simulink model "robot"  (R2022a)
settings: Solver=VariableStepAuto  StartTime=0.0  StopTime=10.0  RelTol=1e-3
undefined symbols (not defined in the file): A, B, C, D, Ki, Kx, l, L
settings Model: Creator=fduterte  LastModifiedBy=Amandine
settings SolverCC: AlgebraicLoopSolver=TrustRegion
settings DebuggingCC: UnconnectedInputMsg=warning  UnconnectedOutputMsg=warning  UnconnectedLineMsg=warning  SFMachineParentedDataDiag=warning
settings RTWCC: DLArmComputeVersion=19.05

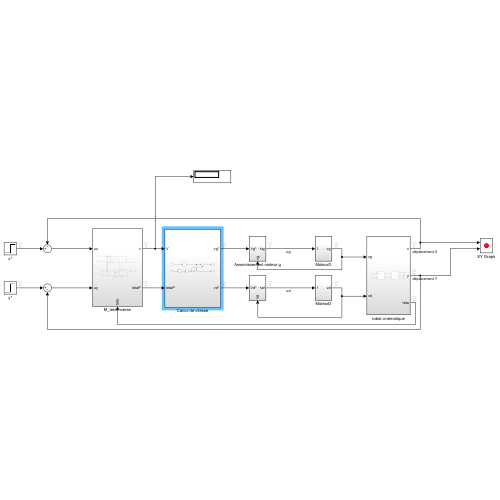
[thumbnail: Simulink's stored preview of the top-level diagram]
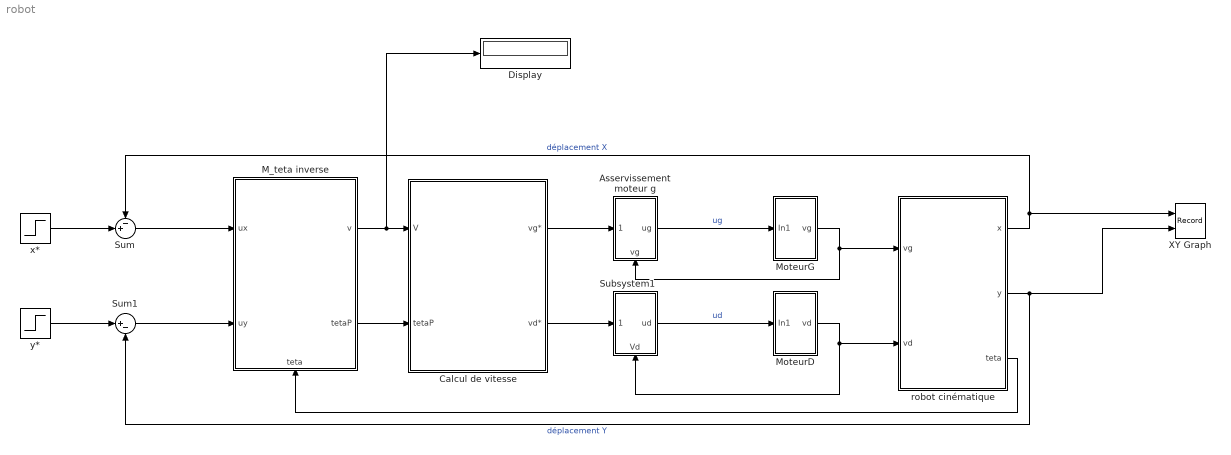
== system robot ==
  Asservissement moteur g : Subsystem
      settings: PortSchema="{\"entries\":[{\"content\":{\"sides\":[{\"content\":{\"connectorIds\":[\"In1\"]},\"type\":\"ConnectorPlacement.EquallySpacedRectSide\",\"uuid\":\"974f67ff-ec86-461c-aa60-533cdeafb118\"},{\"content\":{\"connectorIds\":[\"Out1\"],\"side\":\"RIGHT\"},\"type\":\"ConnectorPlacement.EquallySpacedRectSide\",\"uuid\":\"c8387546-9b25-43fb-a7e6-791e04dec918\"},{\"content\":{\"connectorIds\":[],\"side\":\"TOP\"},\"type\":\"ConnectorPlacement.EquallySpacedRectSide\",\"uuid\":\"89b9c1e4-8a21-45f2-bc89-d00f29d45e47\"},{\"content\":{\"connectorIds\":[\"In2\"],\"side\":\"BOTTOM\"},\"type\":\"ConnectorPlacement.EquallySpacedRectSide\",\"uuid\":\"53d6fe91-d338-4930-b8cd-dea5889de835\"},{\"content\":{\"connectorIds\":[],\"side\":\"HIDDEN\"},\"type\":\"ConnectorPlacement.EquallySpacedRectSide\",\"uuid\":\"29b397e1-e792-4e18-a134-a46f0e718b0f\"}]},\"type\":\"ConnectorPlacement.EquallySpacedConnector\",\"uuid\":\"81d111f1-5eeb-4176-9ac3-35ecafc98cd8\"}],\"packageUris\":[\"http://schema.mathworks.com/mf0/Connector/R2020b\"],\"version\":\"1.0\"}"
  Calcul de vitesse : Subsystem
  Display : Display
  M_teta inverse : Subsystem
      settings: PortSchema="{\"entries\":[{\"content\":{\"sides\":[{\"content\":{\"connectorIds\":[\"In1\",\"In2\"]},\"type\":\"ConnectorPlacement.EquallySpacedRectSide\",\"uuid\":\"46188908-b1cc-4882-9b8e-a8476c333113\"},{\"content\":{\"connectorIds\":[\"Out1\",\"Out2\"],\"side\":\"RIGHT\"},\"type\":\"ConnectorPlacement.EquallySpacedRectSide\",\"uuid\":\"d9e3f140-d678-4bcd-b58f-e0cf2d32dddf\"},{\"content\":{\"connectorIds\":[],\"side\":\"TOP\"},\"type\":\"ConnectorPlacement.EquallySpacedRectSide\",\"uuid\":\"a6a59054-5aa4-4aac-8c2f-440078fd31e6\"},{\"content\":{\"connectorIds\":[\"In3\"],\"side\":\"BOTTOM\"},\"type\":\"ConnectorPlacement.EquallySpacedRectSide\",\"uuid\":\"d37c5d7c-eb10-4efc-bec5-b12ca0db436e\"},{\"content\":{\"connectorIds\":[],\"side\":\"HIDDEN\"},\"type\":\"ConnectorPlacement.EquallySpacedRectSide\",\"uuid\":\"27b7b574-64a3-4ae5-a49b-592b93501c4d\"}]},\"type\":\"ConnectorPlacement.EquallySpacedConnector\",\"uuid\":\"41e6c7f6-3ce7-4034-83c9-1a8b5fe3dc83\"}],\"packageUris\":[\"http://schema.mathworks.com/mf0/Connector/R2020b\"],\"version\":\"1.0\"}"
  MoteurD : Subsystem
  MoteurG : Subsystem
  Subsystem1 : Subsystem
      settings: PortSchema="{\"entries\":[{\"content\":{\"sides\":[{\"content\":{\"connectorIds\":[\"In1\"]},\"type\":\"ConnectorPlacement.EquallySpacedRectSide\",\"uuid\":\"974f67ff-ec86-461c-aa60-533cdeafb118\"},{\"content\":{\"connectorIds\":[\"Out1\"],\"side\":\"RIGHT\"},\"type\":\"ConnectorPlacement.EquallySpacedRectSide\",\"uuid\":\"c8387546-9b25-43fb-a7e6-791e04dec918\"},{\"content\":{\"connectorIds\":[],\"side\":\"TOP\"},\"type\":\"ConnectorPlacement.EquallySpacedRectSide\",\"uuid\":\"89b9c1e4-8a21-45f2-bc89-d00f29d45e47\"},{\"content\":{\"connectorIds\":[\"In2\"],\"side\":\"BOTTOM\"},\"type\":\"ConnectorPlacement.EquallySpacedRectSide\",\"uuid\":\"920a09e2-1f74-455c-9562-9225d36fe6fa\"},{\"content\":{\"connectorIds\":[],\"side\":\"HIDDEN\"},\"type\":\"ConnectorPlacement.EquallySpacedRectSide\",\"uuid\":\"29b397e1-e792-4e18-a134-a46f0e718b0f\"}]},\"type\":\"ConnectorPlacement.EquallySpacedConnector\",\"uuid\":\"81d111f1-5eeb-4176-9ac3-35ecafc98cd8\"}],\"packageUris\":[\"http://schema.mathworks.com/mf0/Connector/R2020b\"],\"version\":\"1.0\"}"
  Sum : Sum  Inputs=-+|
  Sum1 : Sum  Inputs=|+-
  XY Graph : Record  FileSettingsInternal="{\"entries\":[{\"content\":{\"excelSettings\":{\"content\":{},\"type\":\"Streamout.ExcelSettings\"}},\"type\":\"Streamout.FileSettingStorage\",\"uuid\":\"d9b7ccbf-8b1c-4774-986d-cf4be9a417a1\"}],\"packageUris\":[\"http://schema.mathworks.com/mf0/streamout_blocks/R2020a\"],\"version\":\"1.0\"}"  Layout=[1 1]  SignalsInternal="{\"entries\":[{\"content\":{\"signals\":[{\"content\":{\"blockPath\":[\"robot/XY Graph\"],\"channel\":[],\"dimensions\":[1],\"domain\":\"robot/XY Graph\",\"lineColor\":\"#a2142f\",\"plots\":[1],\"port\":1,\"sid\":[],\"signalID\":17,\"signalName\":\"XY Graph:1\"},\"type\":\"RecordBlkView.Signal\",\"uuid\":\"e619f21a-7836-4c61-a051-832b143e0227\"},{\"content\":{\"blockPath\":[\"robot/XY Graph\"],\"channel\":[],\"dimensions\":[1],\"domain\":\"robot/XY Graph\",\"lineColor\":\"#139fff\",\"plots\":[1],\"port\":2,\"sid\":[],\"signalID\":20,\"signalName\":\"XY Graph:2\"},\"type\":\"RecordBlkView.Signal\",\"uuid\":\"4c19a49e-2d7a-439d-9925-7ed591ba5977\"}]},\"type\":\"RecordBlkView.InputSignals\",\"uuid\":\"d8d664c2-0254-4fe2-9c50-e0796b544cb5\"}],\"packageUris\":[\"http://schema.mathworks.com/mf0/streamout_blocks/R2020a\"],\"version\":\"1.0\"}"  VisualizationBindings="{\"xyplotplugin\":{\"info\":[{\"series\":[{\"bindingParametersList\":[{\"parameter\":\"X-Axis\",\"signalID\":17,\"signalName\":\"XY Graph:1\"},{\"parameter\":\"Y-Axis\",\"signalID\":20,\"signalName\":\"XY Graph:2\"}],\"seriesID\":55674}],\"subplotID\":1}]}}"  CompatibilityTag=XY  st=-1
  robot cinématique : Subsystem
  x* : Step  After=1000  SampleTime=0
  y* : Step  After=500  SampleTime=0
  wires:
  x*/1 -> Sum/2
  robot cinématique/2(y) -> XY Graph/2, Sum1/2  "déplacement Y"
  robot cinématique/3(teta) -> M_teta inverse/3(teta)
  Sum1/1 -> M_teta inverse/2(uy)
  robot cinématique/1(x) -> XY Graph/1, Sum/1  "déplacement X"
  Asservissement moteur g/1(ug) -> MoteurG/1(In1)  "ug"
  MoteurG/1(vg) -> robot cinématique/1(vg), Asservissement moteur g/2(vg)
  MoteurD/1(vd) -> robot cinématique/2(vd), Subsystem1/2(Vd)
  Sum/1 -> M_teta inverse/1(ux)
  Subsystem1/1(ud) -> MoteurD/1(In1)  "ud"
  Calcul de vitesse/1(vg*) -> Asservissement moteur g/1(Vg*)
  Calcul de vitesse/2(vd*) -> Subsystem1/1(Vd*)
  M_teta inverse/1(v) -> Display/1, Calcul de vitesse/1(V)
  M_teta inverse/2(tetaP) -> Calcul de vitesse/2(tetaP)
  y*/1 -> Sum1/1

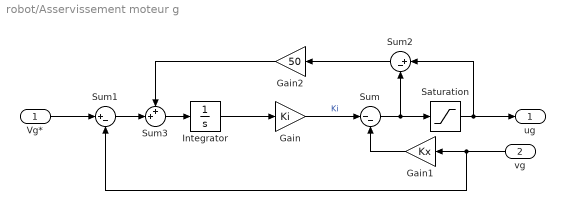
== system robot/Asservissement moteur g ==
  Vg* : Inport
  vg : Inport  Port=2
  Gain : Gain  Gain=Ki
  Gain1 : Gain  Gain=Kx
  Gain2 : Gain  Gain=50
  Integrator : Integrator
  Saturation : Saturate  UpperLimit=9  LowerLimit=-9
  Sum : Sum  Inputs=|--
  Sum1 : Sum  Inputs=|+-
  Sum2 : Sum  Inputs=|+-
  Sum3 : Sum  Inputs=++|
  ug : Outport
  wires:
  Integrator/1 -> Gain/1
  Gain/1 -> Sum/1  "Ki"
  Vg*/1 -> Sum1/1
  Gain1/1 -> Sum/2
  vg/1 -> Sum1/2, Gain1/1
  Sum1/1 -> Sum3/2
  Sum3/1 -> Integrator/1
  Sum2/1 -> Gain2/1
  Saturation/1 -> Sum2/1, ug/1
  Sum/1 -> Sum2/2, Saturation/1
  Gain2/1 -> Sum3/1

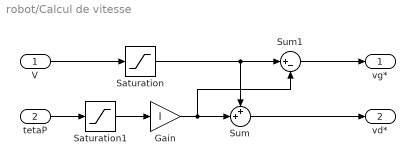
== system robot/Calcul de vitesse ==
  V : Inport
  tetaP : Inport  Port=2
  Gain : Gain  Gain=l
  Saturation : Saturate  UpperLimit=300  LowerLimit=-300
  Saturation1 : Saturate  UpperLimit=300/l  LowerLimit=-300/l
  Sum : Sum  Inputs=++|
  Sum1 : Sum  Inputs=|+-
  vg* : Outport
  vd* : Outport  Port=2
  wires:
  tetaP/1 -> Saturation1/1
  V/1 -> Saturation/1
  Gain/1 -> Sum1/2, Sum/2
  Sum/1 -> vd*/1
  Sum1/1 -> vg*/1
  Saturation/1 -> Sum1/1, Sum/1
  Saturation1/1 -> Gain/1

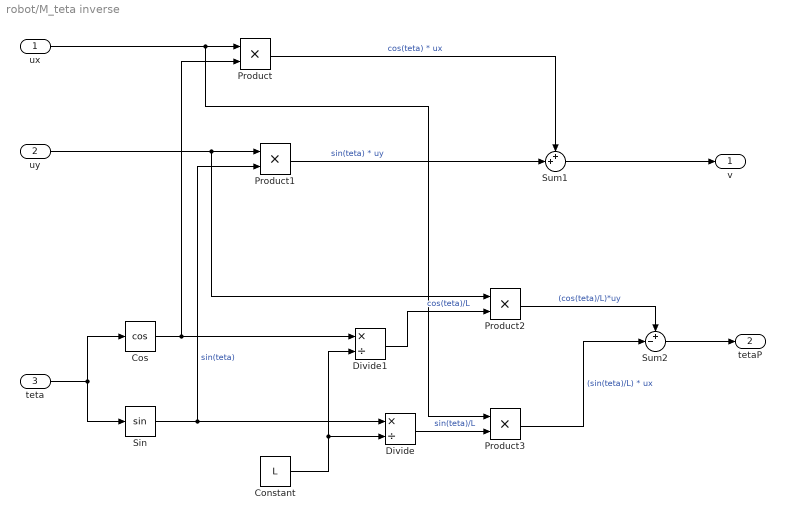
== system robot/M_teta inverse ==
  ux : Inport
  uy : Inport  Port=2
  teta : Inport  Port=3
  Constant : Constant  Value=L
  Cos : Trigonometry  Operator=cos
  Divide : Product  Inputs=*/
  Divide1 : Product  Inputs=*/
  Product{,1..3} (4 alike) : Product
  Sin : Trigonometry
  Sum1 : Sum  Inputs=++|
  Sum2 : Sum  Inputs=+-|
  v : Outport
  tetaP : Outport  Port=2
  wires:
  teta/1 -> Cos/1, Sin/1
  Cos/1 -> Product/2, Divide1/1
  Product1/1 -> Sum1/2  "sin(teta) * uy"
  Sum2/1 -> tetaP/1
  Sum1/1 -> v/1
  ux/1 -> Product3/1, Product/1
  Product/1 -> Sum1/1  "cos(teta) * ux"
  uy/1 -> Product2/1, Product1/1
  Sin/1 -> Divide/1, Product1/2  "sin(teta)"
  Constant/1 -> Divide1/2, Divide/2
  Divide1/1 -> Product2/2  "cos(teta)/L"
  Divide/1 -> Product3/2  "sin(teta)/L"
  Product3/1 -> Sum2/2  "(sin(teta)/L) * ux"
  Product2/1 -> Sum2/1  "(cos(teta)/L)*uy"

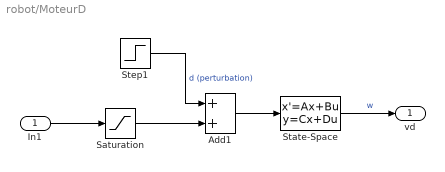
== system robot/MoteurD ==
  In1 : Inport
  Add1 : Sum
  Saturation : Saturate  UpperLimit=9  LowerLimit=-9
  State-Space : StateSpace  A=A  B=B  C=C  D=D  InitialCondition=0
  Step1 : Step  Time=5  After=0  SampleTime=0
  vd : Outport
  wires:
  Step1/1 -> Add1/1  "d (perturbation)"
  Add1/1 -> State-Space/1
  In1/1 -> Saturation/1
  State-Space/1 -> vd/1  "w"
  Saturation/1 -> Add1/2

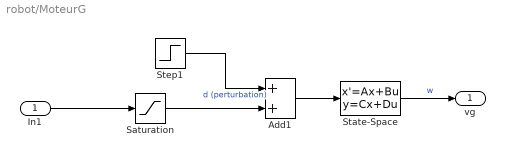
== system robot/MoteurG ==
  In1 : Inport
  Add1 : Sum
  Saturation : Saturate  UpperLimit=9  LowerLimit=-9
  State-Space : StateSpace  A=A  B=B  C=C  D=D  InitialCondition=0
  Step1 : Step  Time=5  After=0  SampleTime=0
  vg : Outport
  wires:
  Step1/1 -> Add1/1  "d (perturbation)"
  Add1/1 -> State-Space/1
  In1/1 -> Saturation/1
  State-Space/1 -> vg/1  "w"
  Saturation/1 -> Add1/2

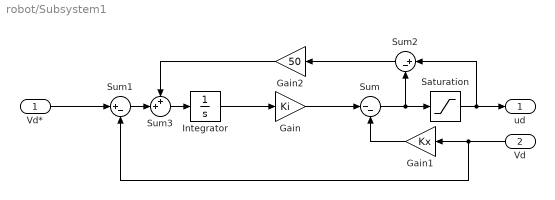
== system robot/Subsystem1 ==
  Vd* : Inport
  Vd : Inport  Port=2
  Gain : Gain  Gain=Ki
  Gain1 : Gain  Gain=Kx
  Gain2 : Gain  Gain=50
  Integrator : Integrator
  Saturation : Saturate  UpperLimit=9  LowerLimit=-9
  Sum : Sum  Inputs=|--
  Sum1 : Sum  Inputs=|+-
  Sum2 : Sum  Inputs=|+-
  Sum3 : Sum  Inputs=++|
  ud : Outport
  wires:
  Integrator/1 -> Gain/1
  Gain/1 -> Sum/1
  Vd*/1 -> Sum1/1
  Gain1/1 -> Sum/2
  Vd/1 -> Sum1/2, Gain1/1
  Sum1/1 -> Sum3/2
  Sum3/1 -> Integrator/1
  Sum2/1 -> Gain2/1
  Sum/1 -> Sum2/2, Saturation/1
  Saturation/1 -> Sum2/1, ud/1
  Gain2/1 -> Sum3/1

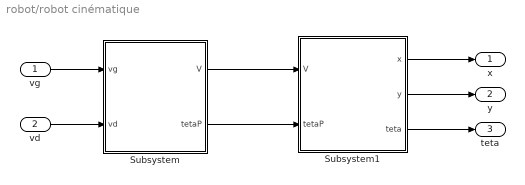
== system robot/robot cinématique ==
  vg : Inport
  vd : Inport  Port=2
  Subsystem : Subsystem
  Subsystem1 : Subsystem
  x : Outport
  y : Outport  Port=2
  teta : Outport  Port=3
  wires:
  Subsystem1/2(y) -> y/1
  Subsystem1/1(x) -> x/1
  Subsystem1/3(teta) -> teta/1
  Subsystem/1(V) -> Subsystem1/1(V)
  Subsystem/2(tetaP) -> Subsystem1/2(tetaP)
  vd/1 -> Subsystem/2(vd)
  vg/1 -> Subsystem/1(vg)

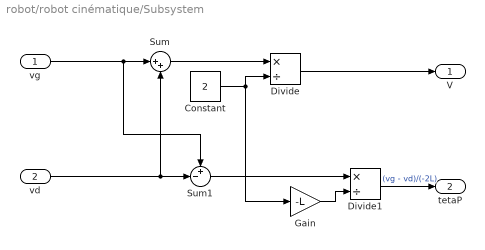
== system robot/robot cinématique/Subsystem ==
  vg : Inport
  vd : Inport  Port=2
  Constant : Constant  Value=2
  Divide : Product  Inputs=*/
  Divide1 : Product  Inputs=*/
  Gain : Gain  Gain=-L
  Sum : Sum  Inputs=|++
  Sum1 : Sum  Inputs=+-|
  V : Outport
  tetaP : Outport  Port=2
  wires:
  vg/1 -> Sum1/1, Sum/1
  vd/1 -> Sum1/2, Sum/2
  Sum/1 -> Divide/1
  Constant/1 -> Gain/1, Divide/2
  Divide/1 -> V/1
  Sum1/1 -> Divide1/1
  Divide1/1 -> tetaP/1  "(vg - vd)/(-2L)"
  Gain/1 -> Divide1/2

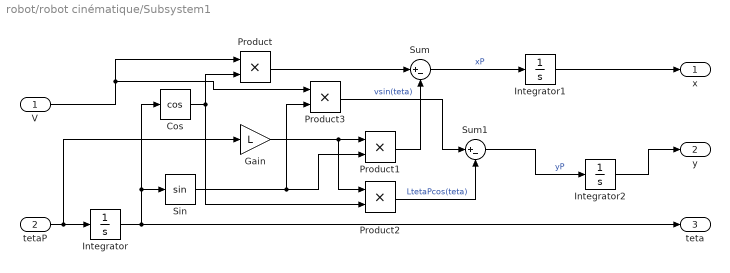
== system robot/robot cinématique/Subsystem1 ==
  V : Inport
  tetaP : Inport  Port=2
  Cos : Trigonometry  Operator=cos
  Gain : Gain  Gain=L
  Integrator : Integrator
  Integrator1 : Integrator
  Integrator2 : Integrator
  Product{,1..3} (4 alike) : Product
  Sin : Trigonometry
  Sum : Sum  Inputs=|+-
  Sum1 : Sum  Inputs=|+-
  x : Outport
  y : Outport  Port=2
  teta : Outport  Port=3
  wires:
  Integrator/1 -> teta/1, Sin/1, Cos/1
  tetaP/1 -> Integrator/1, Gain/1
  V/1 -> Product/1, Product3/1
  Cos/1 -> Product2/2, Product/2
  Product/1 -> Sum/1
  Gain/1 -> Product2/1, Product1/1
  Sin/1 -> Product3/2, Product1/2
  Product1/1 -> Sum/2
  Sum/1 -> Integrator1/1  "xP"
  Product2/1 -> Sum1/2  "LtetaPcos(teta)"
  Sum1/1 -> Integrator2/1  "yP"
  Product3/1 -> Sum1/1  "vsin(teta)"
  Integrator1/1 -> x/1
  Integrator2/1 -> y/1
